simulink library "PiCar_library"  (R2018a)
settings: Solver=VariableStepAuto  StartTime=0.0  StopTime=10.0  RelTol=1e-3
undefined symbols (not defined in the file or in its folder): gray
libraries: visiontextngfix x2, visiontransforms x2, simulink x1, visionanalysis x1, visionstatistics x1, embdlinuxlib x1
settings Model: Creator=Malte  LastModifiedBy=Herib

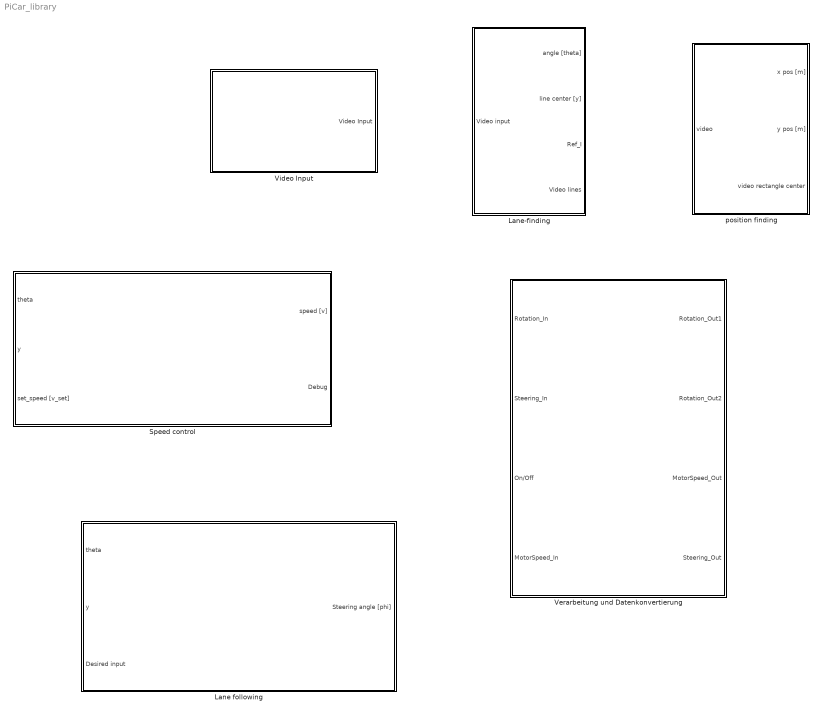
== system PiCar_library ==
  Lane following : Subsystem
  Lane-finding : Subsystem
  Speed control : Subsystem
  Verarbeitung und Datenkonvertierung : Subsystem
  Video Input : Subsystem
  position finding : Subsystem

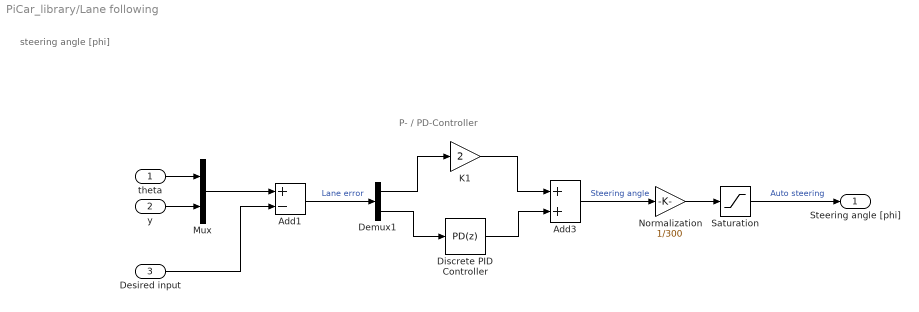
== system PiCar_library/Lane following ==
  note: P- / PD-Controller
  note: steering angle [phi]
  theta : Inport
  y : Inport  Port=2
  Desired input : Inport  Port=3
  Add1 : Sum  Inputs=+-
  Add3 : Sum
  Demux1 : Demux  Outputs=2
  Discrete PID Controller : simulink/Continuous/PID Controller  Controller=PD  TimeDomain=Discrete-time  SampleTime=-1  IntegratorMethod=Forward Euler  FilterMethod=Forward Euler  Form=Parallel  UseFilter=off  ControllerParametersSource=internal  P=18  I=1.5  D=2  N=100  InitialConditionSource=internal  InitialConditionForIntegrator=0  InitialConditionForFilter=0  ExternalReset=none  LimitOutput=off  UpperSaturationLimit=inf  LowerSaturationLimit=-inf  LinearizeAsGain=off  AntiWindupMode=none  Kb=1  TrackingMode=off  Kt=1  PParamMin=[]  PParamMax=[]  IParamMin=[]  IParamMax=[]  DParamMin=[]  DParamMax=[]  NParamMin=[]  NParamMax=[]  KbParamMin=[]  KbParamMax=[]  KtParamMin=[]  KtParamMax=[]  POutMin=[]  POutMax=[]  IOutMin=[]  IOutMax=[]  DOutMin=[]  DOutMax=[]  NOutMin=[]  NOutMax=[]  KbOutMin=[]  KbOutMax=[]  KtOutMin=[]  KtOutMax=[]  IntegratorOutMin=[]  IntegratorOutMax=[]  FilterOutMin=[]  FilterOutMax=[]  SumOutMin=[]  SumOutMax=[]  SumI1OutMin=[]  SumI1OutMax=[]  SumI2OutMin=[]  SumI2OutMax=[]  SumI3OutMin=[]  SumI3OutMax=[]  SumDOutMin=[]  SumDOutMax=[]  SaturationOutMin=[]  SaturationOutMax=[]  IntegratorContinuousStateAttributes=''  IntegratorStateMustResolveToSignalObject=off  IntegratorRTWStateStorageClass=Auto  FilterContinuousStateAttributes=''  FilterStateMustResolveToSignalObject=off  FilterRTWStateStorageClass=Auto  DifferentiatorICPrevScaledInput=0  DifferentiatorOutMin=[]  DifferentiatorOutMax=[]  FilterDiffOutCoefMin=[]  FilterDiffOutCoefMax=[]  SumDenOutMin=[]  SumDenOutMax=[]  SumNumOutMin=[]  SumNumOutMax=[]  ReciprocalOutMin=[]  ReciprocalOutMax=[]  DivideOutMin=[]  DivideOutMax=[]  TunerSelectOption=Transfer Function Based (PID Tuner App)
  K1 : Gain  Gain=2
  Mux : Mux  Inputs=2
  Normalization : Gain  Gain=1/300
  Saturation : Saturate  UpperLimit=1  LowerLimit=-1
  Steering angle [phi] : Outport
  wires:
  K1/1 -> Add3/1
  Demux1/1 -> K1/1
  Add1/1 -> Demux1/1  "Lane error"
  Demux1/2 -> Discrete PID Controller/1
  Discrete PID Controller/1 -> Add3/2
  Add3/1 -> Normalization/1  "Steering angle"
  Saturation/1 -> Steering angle [phi]/1  "Auto steering"
  Normalization/1 -> Saturation/1
  Desired input/1 -> Add1/2
  Mux/1 -> Add1/1
  y/1 -> Mux/2
  theta/1 -> Mux/1

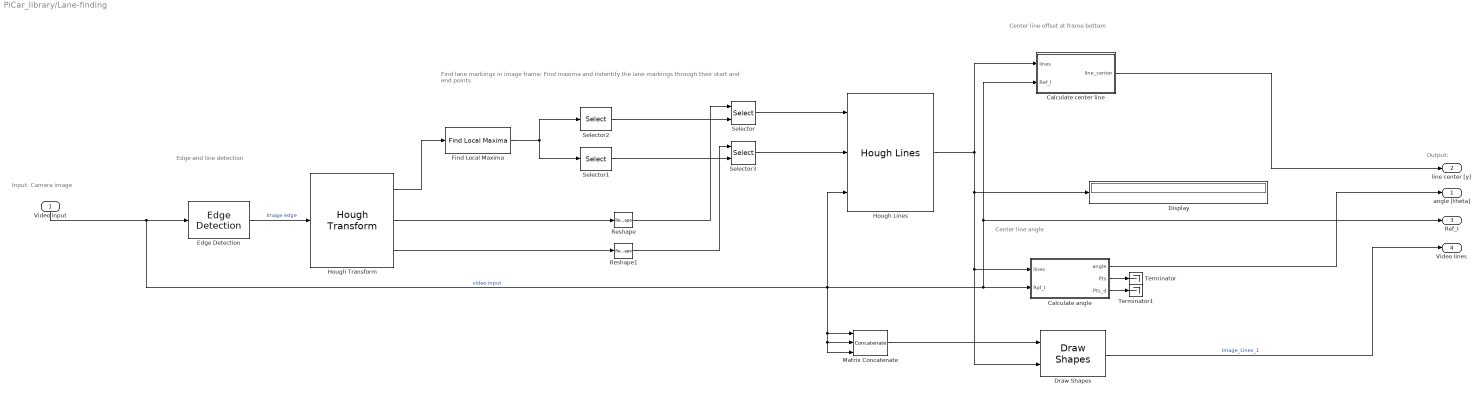
== system PiCar_library/Lane-finding ==
  note: Center line offset at frame bottom
  note: Center line angle
  note: Find lane markings in image frame:
      | Find maxima and indentify the lane markings through their start and end points
  note: Edge and line detection
  note: Input: Camera image
  note: Output:
  Video input : Inport
  Calculate angle : MATLAB Function  TreatAsAtomicUnit=on
  Calculate center line : MATLAB Function  TreatAsAtomicUnit=on
  Display : Display
  Draw Shapes : visiontextngfix/Draw Shapes  shape=Lines  fill=off  lineWidth=1  fillClrSource=Specify via dialog  display=User-specified value  intensity=200  color=[0 0 255]  opacity=0.6  viewport=Entire image  antialiasing=off  inType=Obsolete  imagePorts=One multidimensional signal  prodOutputMode=Binary point scaling  prodOutputWordLength=32  prodOutputFracLength=14  memoryMode=Specify word length  memoryWordLength=16  memoryFracLength=14  roundingMode=Floor  overflowMode=off
      settings: SourceProductName=Computer Vision System Toolbox
  Edge Detection : visionanalysis/Edge Detection  method=Sobel  outputType=Binary image  userDefinedThreshold=off  thresholdSource=Input port  threshold=20  thresholdTuning=4  edgeThinning=off  threshold_canny=[0.25 0.60]  autoPercent=70  sigma=1  roundingMode=Floor  overflowMode=off  prodOutputMode=Binary point scaling  prodOutputWordLength=32  prodOutputFracLength=8  prodOutputSlope=2^-8  accumSlope=2^-8  outputSlope=2^-4
      settings: SourceProductName=Computer Vision System Toolbox  SourceProductBaseCode=VP
  Find Local Maxima : visionstatistics/Find Local Maxima  num_peaks=2  nhood_size=[5 7]  src_thresh=Obsolete9b  src_thresh_inuse=Specify via dialog  threshold=10  inputIsHough=off  dt_peak=uint32  isOutVarDim=on  dt_count=uint32
      settings: SourceProductName=Computer Vision System Toolbox  SourceProductBaseCode=VP
  Hough Lines : visiontransforms/Hough Lines  sineCompMethod=Trigonometric function  thetaRes=pi/180  firstCoeffMode=Specify word length  firstCoeffWordLength=16  firstCoeffFracLength=15  prodOutputMode=Binary point scaling  prodOutputWordLength=32  prodOutputFracLength=16  roundingMode=Nearest  overflowMode=on
      settings: SourceProductName=Computer Vision System Toolbox  SourceProductBaseCode=VP
  Hough Transform : visiontransforms/Hough Transform  theta_res=pi/180  rho_res=1  out_theta_rho=on  outdtmode=double  firstCoeffMode=Binary point scaling  firstCoeffWordLength=16  firstCoeffFracLength=14  secondCoeffMode=Binary point scaling  secondCoeffWordLength=32  secondCoeffFracLength=16  outputMode=Binary point scaling  outputWordLength=16  outputFracLength=0  accumMode=Binary point scaling  accumWordLength=32  accumFracLength=20  prodOutputMode=Binary point scaling  prodOutputWordLength=32  prodOutputFracLength=20  memoryMode=Binary point scaling  memoryWordLength=32  memoryFracLength=16  roundingMode=Nearest  overflowMode=on
      settings: SourceProductName=Computer Vision System Toolbox  SourceProductBaseCode=VP
  Matrix Concatenate : Concatenate  NumInputs=3  Mode=Multidimensional array  ConcatenateDimension=3
  Reshape : Reshape
  Reshape1 : Reshape
  Selector : Selector  IndexOptions=Index vector (port)  Indices=[1 3]  OutputSizes=1
  Selector1 : Selector  NumberOfDimensions=2  InputPortWidth=3  IndexOptions=Select all,Index vector (dialog)  Indices=[1 3],2  OutputSizes=1,1
  Selector2 : Selector  NumberOfDimensions=2  InputPortWidth=3  IndexOptions=Select all,Index vector (dialog)  Indices=[1 3],1  OutputSizes=1,1
  Selector3 : Selector  IndexOptions=Index vector (port)  Indices=[1 3]  OutputSizes=1
  Terminator : Terminator
  Terminator1 : Terminator
  angle [theta] : Outport
  line center [y] : Outport  Port=2
  Ref_I : Outport  Port=3
  Video lines : Outport  Port=4
  wires:
  Calculate angle/2(Pts) -> Terminator/1
  Calculate angle/3(Pts_d) -> Terminator1/1
  Edge Detection/1 -> Hough Transform/1  "Image edge"
  Video input/1 -> Calculate angle/2(Ref_I), Calculate center line/2(Ref_I), Ref_I/1, Hough Lines/3, Matrix Concatenate/1, Matrix Concatenate/2, Matrix Concatenate/3, Edge Detection/1  "video input"
  Hough Transform/2 -> Reshape/1
  Hough Transform/3 -> Reshape1/1
  Hough Transform/1 -> Find Local Maxima/1
  Selector1/1 -> Selector3/2
  Selector2/1 -> Selector/2
  Find Local Maxima/1 -> Selector2/1, Selector1/1
  Selector/1 -> Hough Lines/1
  Reshape/1 -> Selector/1
  Selector3/1 -> Hough Lines/2
  Reshape1/1 -> Selector3/1
  Matrix Concatenate/1 -> Draw Shapes/1
  Calculate angle/1(angle) -> angle [theta]/1
  Draw Shapes/1 -> Video lines/1  "Image_Lines_1"
  Hough Lines/1 -> Calculate center line/1(lines), Display/1, Draw Shapes/2, Calculate angle/1(lines)
  Calculate center line/1(line_center) -> line center [y]/1

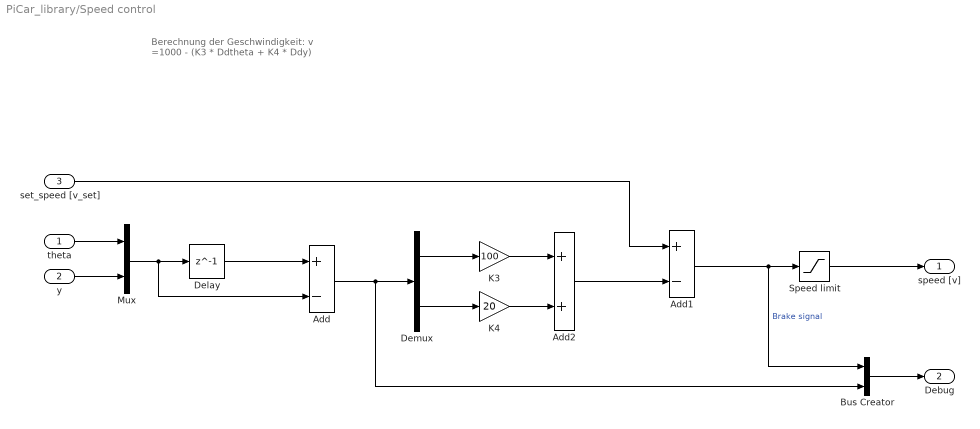
== system PiCar_library/Speed control ==
  note: Berechnung der Geschwindigkeit:
      |
      | v =1000 - (K3 * Ddtheta + K4 * Ddy)
  theta : Inport
  y : Inport  Port=2
  set_speed [v_set] : Inport  Port=3
  Add : Sum  Inputs=+-
  Add1 : Sum  Inputs=+-
  Add2 : Sum
  Bus Creator : BusCreator  Inputs=2
  Delay : Delay  DelayLength=1  InitialCondition=0
  Demux : Demux  Outputs=2
  K3 : Gain  Gain=100
  K4 : Gain  Gain=20
  Mux : Mux  Inputs=2
  Speed limit : Saturate  UpperLimit=0.4  LowerLimit=0
  speed [v] : Outport
  Debug : Outport  Port=2
  wires:
  Mux/1 -> Add/2, Delay/1
  Delay/1 -> Add/1
  Add/1 -> Bus Creator/2, Demux/1
  Demux/1 -> K3/1
  Demux/2 -> K4/1
  Add2/1 -> Add1/2
  Add1/1 -> Bus Creator/1, Speed limit/1  "Brake signal"
  set_speed [v_set]/1 -> Add1/1
  K4/1 -> Add2/2
  K3/1 -> Add2/1
  Bus Creator/1 -> Debug/1
  y/1 -> Mux/2
  theta/1 -> Mux/1
  Speed limit/1 -> speed [v]/1

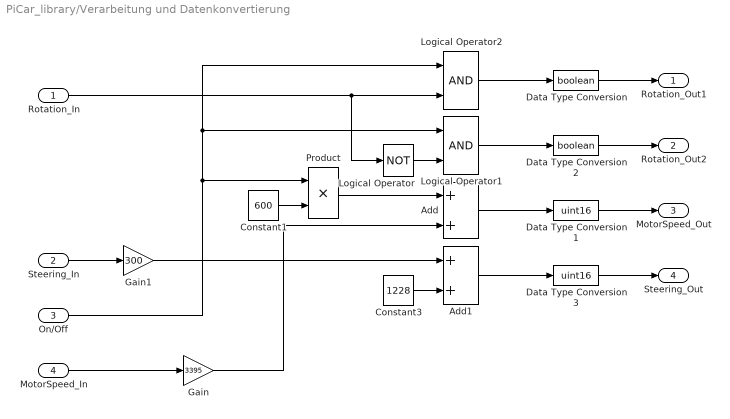
== system PiCar_library/Verarbeitung und Datenkonvertierung ==
  Rotation_In : Inport
  Steering_In : Inport  Port=2
  On/Off : Inport  Port=3
  MotorSpeed_In : Inport  Port=4
  Add : Sum
  Add1 : Sum
  Constant1 : Constant  Value=600
  Constant3 : Constant  Value=1228  OutMin=819  OutMax=1638
  Data Type Conversion : DataTypeConversion  OutDataTypeStr=boolean
  Data Type Conversion1 : DataTypeConversion  OutDataTypeStr=uint16
  Data Type Conversion2 : DataTypeConversion  OutDataTypeStr=boolean
  Data Type Conversion3 : DataTypeConversion  OutDataTypeStr=uint16
  Gain : Gain  Gain=3395
  Gain1 : Gain  Gain=300
  Logical Operator : Logic  Operator=NOT  AllPortsSameDT=off  OutDataTypeStr=boolean
  Logical Operator1 : Logic  AllPortsSameDT=off  OutDataTypeStr=boolean
  Logical Operator2 : Logic  AllPortsSameDT=off  OutDataTypeStr=boolean
  Product : Product
  Rotation_Out1 : Outport
  Rotation_Out2 : Outport  Port=2
  MotorSpeed_Out : Outport  Port=3
  Steering_Out : Outport  Port=4
  wires:
  Logical Operator1/1 -> Data Type Conversion2/1
  Logical Operator2/1 -> Data Type Conversion/1
  Logical Operator/1 -> Logical Operator1/2
  On/Off/1 -> Logical Operator1/1, Logical Operator2/1, Product/1
  Constant3/1 -> Add1/2
  Rotation_In/1 -> Logical Operator/1, Logical Operator2/2
  Add/1 -> Data Type Conversion1/1
  Add1/1 -> Data Type Conversion3/1
  Constant1/1 -> Product/2
  Product/1 -> Add/1
  Data Type Conversion1/1 -> MotorSpeed_Out/1
  Data Type Conversion3/1 -> Steering_Out/1
  Data Type Conversion2/1 -> Rotation_Out2/1
  MotorSpeed_In/1 -> Gain/1
  Data Type Conversion/1 -> Rotation_Out1/1
  Steering_In/1 -> Gain1/1
  Gain/1 -> Add/2
  Gain1/1 -> Add1/1

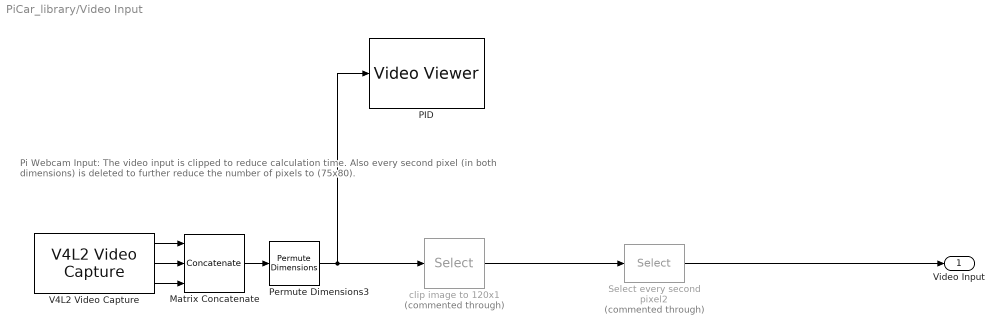
== system PiCar_library/Video Input ==
  note: Pi Webcam Input:
      | The video input is clipped to reduce calculation time. Also every second pixel (in both dimensions) is deleted to further reduce the number of pixels
      | to (75x80).
  Matrix Concatenate : Concatenate  NumInputs=3  Mode=Multidimensional array  ConcatenateDimension=3
  PID : VideoViewer  colormapValue=gray(256)  FigPos=[1 1038 1920 938]  OpenAtMdlStart=off
  Permute Dimensions3 : PermuteDimensions  Order=[2,1,3]
  Select every second pixel2 : Selector  Commented=through  NumberOfDimensions=2  InputPortWidth=3  IndexOptions=Select all,Index vector (dialog)  Indices=[1:2:80],[1:2:160]  OutputSizes=1,1
  V4L2 Video Capture : embdlinuxlib/V4L2 Video Capture  m_devName='/dev/video0'  roi=[0, 0, 640, 480]  imSizeSelection=320x240  imSize=[640, 480]  pixelFormat=RGB  pixelOrder=Planar  sampleTime=1/10  simOutput=Colorbars  blockPlatform=Raspberry Pi
      settings: SourceProductName=Simulink Support Package for Raspberry Pi Hardware  SourceProductBaseCode=RASPPI
  clip image to 120x1 : Selector  Commented=through  NumberOfDimensions=2  InputPortWidth=3  IndexOptions=Index vector (dialog),Index vector (dialog)  Indices=[150:1:210],[1:2:320]  OutputSizes=1,1
  Video Input : Outport
  wires:
  Permute Dimensions3/1 -> PID/1, clip image to 120x1/1
  clip image to 120x1/1 -> Select every second pixel2/1
  V4L2 Video Capture/2 -> Matrix Concatenate/2
  V4L2 Video Capture/3 -> Matrix Concatenate/3
  Select every second pixel2/1 -> Video Input/1
  V4L2 Video Capture/1 -> Matrix Concatenate/1
  Matrix Concatenate/1 -> Permute Dimensions3/1

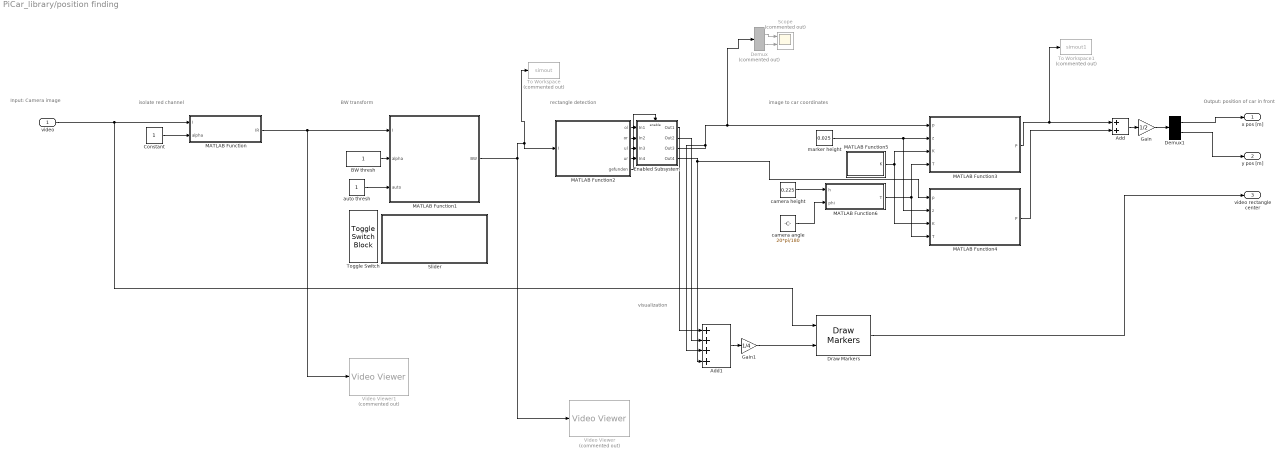
== system PiCar_library/position finding ==
  note: Input: Camera image
  note: Output: position of car in front
  note: isolate red channel
  note: BW transform
  note: rectangle detection
  note: image to car coordinates
  note: visualization
  video : Inport
  Add : Sum  Inputs=2
  Add1 : Sum  Inputs=4
  BW thresh : Constant
  Constant : Constant
  Demux : Demux  Commented=on  Outputs=2
  Demux1 : Demux  Outputs=2
  Draw Markers : visiontextngfix/Draw Markers  shape=Circle  size=3  fill=off  fillClrSource=Specify via dialog  display=Black  intensity=200  color=[200 255 100]  opacity=0.6  viewport=Entire image  antialiasing=off  inType=Obsolete  imagePorts=One multidimensional signal  prodOutputMode=Binary point scaling  prodOutputWordLength=32  prodOutputFracLength=14  memoryMode=Specify word length  memoryWordLength=16  memoryFracLength=15  roundingMode=Floor  overflowMode=off
      settings: SourceProductName=Computer Vision System Toolbox  SourceProductBaseCode=VP
  Enabled Subsystem : Subsystem  TreatAsAtomicUnit=on
  Gain : Gain  Gain=1/2
  Gain1 : Gain  Gain=1/4
  MATLAB Function : MATLAB Function  TreatAsAtomicUnit=on
  MATLAB Function1 : MATLAB Function  TreatAsAtomicUnit=on
  MATLAB Function2 : MATLAB Function  TreatAsAtomicUnit=on
  MATLAB Function3 : MATLAB Function  TreatAsAtomicUnit=on
  MATLAB Function4 : MATLAB Function  TreatAsAtomicUnit=on
  MATLAB Function5 : MATLAB Function  TreatAsAtomicUnit=on
  MATLAB Function6 : MATLAB Function  TreatAsAtomicUnit=on
  Scope : Scope  Commented=on  NumInputPorts=2
  Slider : Subsystem  DialogController=hmiCreateDDGDialog  IsWebBlock=on  mask(MWDashboardBlock){webBlockId=af7e4ece-416e-4c7c-9f64-5e96a6a09053, webBlockType=slider, ShowInLibBrowser=on, ShowInitialText=on, HMISrcModelName=PiCar_library}
      mask prompts: webBlockId "WebBlock Id"; webBlockType "WebBlock Type"; HMISrcModelName "Source Model"
      mask help: SimulinkHMI:dialogs:SliderDialogDesc
      mask Help: helpview([docroot '/mapfiles/simulink.map'], 'hmi_slider')
      mask Display:
      | if strcmp(get_param(bdroot(gcb),'BlockDiagramType'), 'library')
      |     image([(matlabroot) '/toolbox/simulink/hmi/icons/Slider.png']);
      | end
  To Workspace : ToWorkspace  Commented=on  VariableName=simout  SaveFormat=Structure  SampleTime=-1
      settings: MaxDataPoints=1
  To Workspace1 : ToWorkspace  Commented=on  VariableName=simout1  SaveFormat=Timeseries  SampleTime=-1
  Toggle Switch : ToggleSwitchBlock  WebBlockId=151
      settings: Values={{'Off', 'On'}, [0 1]}
  Video Viewer : VideoViewer  Commented=on  FigPos=[2041 741 418 304]
  Video Viewer1 : VideoViewer  Commented=on  FigPos=[2041 741 418 304]
  auto thresh : Constant
  camera angle : Constant  Value=20*pi/180
  camera height : Constant  Value=0.225
  marker height : Constant  Value=0.025
  x pos [m] : Outport
  y pos [m] : Outport  Port=2
  video rectangle center : Outport  Port=3
  wires:
  Constant/1 -> MATLAB Function/2(alpha)
  MATLAB Function/1(IR) -> Video Viewer1/1, MATLAB Function1/1(I)
  BW thresh/1 -> MATLAB Function1/2(alpha)
  auto thresh/1 -> MATLAB Function1/3(auto)
  MATLAB Function1/1(BW) -> To Workspace/1, MATLAB Function2/1(I), Video Viewer/1
  MATLAB Function3/1(P) -> To Workspace1/1, Add/1
  Add/1 -> Gain/1
  Add1/1 -> Gain1/1
  Enabled Subsystem/1(Out1) -> Add1/1
  Enabled Subsystem/2(Out2) -> Add1/2
  Gain1/1 -> Draw Markers/2
  video/1 -> Draw Markers/1, MATLAB Function/1(I)
  Draw Markers/1 -> video rectangle center/1
  MATLAB Function4/1(P) -> Add/2
  marker height/1 -> MATLAB Function4/2(z), MATLAB Function3/2(z)
  MATLAB Function5/1(K) -> MATLAB Function4/3(K), MATLAB Function3/3(K)
  MATLAB Function6/1(T) -> MATLAB Function4/4(T), MATLAB Function3/4(T)
  camera height/1 -> MATLAB Function6/1(h)
  camera angle/1 -> MATLAB Function6/2(phi)
  Demux1/1 -> x pos [m]/1
  MATLAB Function2/5(gefunden) -> Enabled Subsystem/Enable
  MATLAB Function2/1(ol) -> Enabled Subsystem/1(In1)
  MATLAB Function2/2(or) -> Enabled Subsystem/2(In2)
  MATLAB Function2/3(ul) -> Enabled Subsystem/3(In3)
  MATLAB Function2/4(ur) -> Enabled Subsystem/4(In4)
  Demux/2 -> Scope/2
  Demux/1 -> Scope/1
  Enabled Subsystem/3(Out3) -> MATLAB Function3/1(p), Demux/1, Add1/3
  Enabled Subsystem/4(Out4) -> MATLAB Function4/1(p), Add1/4
  Gain/1 -> Demux1/1
  Demux1/2 -> y pos [m]/1

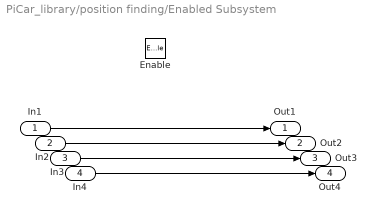
== system PiCar_library/position finding/Enabled Subsystem ==
  In1 : Inport
  In2 : Inport  Port=2
  In3 : Inport  Port=3
  In4 : Inport  Port=4
  Enable : EnablePort  StatesWhenEnabling=reset  PropagateVarSize=During execution
  Out1 : Outport
  Out2 : Outport  Port=2
  Out3 : Outport  Port=3
  Out4 : Outport  Port=4
  wires:
  In1/1 -> Out1/1
  In2/1 -> Out2/1
  In3/1 -> Out3/1
  In4/1 -> Out4/1

== system PiCar_library/position finding/Slider ==

== matlab function PiCar_library/Lane-finding/Calculate angle ==
  data: lines input; angle output; Pts output; Pts_d output; Ref_I input
function [angle, Pts, Pts_d] = angle(lines, Ref_I)

IMAGE_SIZE = size(Ref_I);
IMAGE_HEIGHT = IMAGE_SIZE(1);
IMAGE_WIDTH = IMAGE_SIZE(2);
points = zeros(2,4);

% Sorting the lines
if double(lines(1,1)) < double(lines(2,1))
    points(1,:) = lines(1,:);
    points(2,:) = lines(2,:);
else
    points(1,:) = lines(2,:);
    points(2,:) = lines(1,:);
end

% Calculate the lane center, top and bottom
x_center = double((points(1,:) + points(2,:))/2);

% Calculate the angle of the centerline: 0 -> vertical
angle = atan((x_center(3) - x_center(1))/IMAGE_HEIGHT);

% Auxilliary lines
Pts = int32([x_center(1), 1, x_center(3), 75]);
Pts_d = int32([IMAGE_WIDTH/2, 1, IMAGE_WIDTH/2, 75]);

% angles = atan2d(double((lines(:,1) - lines(:,3))), -double(lines(:,2) - lines(:,4)));

== matlab function PiCar_library/Lane-finding/Calculate center line ==
  data: lines input; line_center output; Ref_I input
function line_center = center(lines, Ref_I)

IMAGE_SIZE = size(Ref_I);
IMAGE_HEIGHT = IMAGE_SIZE(1);
IMAGE_WIDTH = IMAGE_SIZE(2);
points = zeros(2,4);

% Sorting the lines
if double(lines(1,1)) < double(lines(2,1))
    points(1,:) = lines(1,:);
    points(2,:) = lines(2,:);
else
    points(1,:) = lines(2,:);
    points(2,:) = lines(1,:);
end

% Calculate the lane center, top and bottom
x_center = double((points(1,:) + points(2,:))/2);

% Output the lane center at the bottom of the picture
line_center = x_center(3);

== matlab function PiCar_library/position finding/MATLAB Function ==
  data: I input; IR output; alpha input
function IR = isolate_red(I, alpha)
    IR = I(:,:,1) - alpha*I(:,:,2) - alpha*I(:,:,3);
end

== matlab function PiCar_library/position finding/MATLAB Function1 ==
  data: I input; BW output; alpha input; auto input
function BW = BW_im(I, alpha, auto)
    if(auto)
        BW = imbinarize(I);
    else
        BW = imbinarize(I,alpha);
    end
end

== matlab function PiCar_library/position finding/MATLAB Function2 ==
  data: I input; ol output; or output; ul output; ur output; gefunden output
function [ol, or, ul, ur, gefunden]  = finderechteck(I)
%fuer die Aufloesung 160x120
%findet koordinaten der Ecken des rechteckes im Bild
%IGr=rgb2gray(I);
%IG=imgaussfilt(IGr,5);
%I=max(I(:,:,1),0); %rot vorheben
%imshow([I(:,:,1) I(:,:,2); I(:,:,3) I(:,:,1)-0.5*I(:,:,2)-0.5*I(:,:,3)]);
%imshow(I);
x1=floor(size(I,2)/2);
y1=floor(size(I,1)/2);
iteration=1;
schrittgroesse=10;
%imshow(I)
%hold on;
finished=false;
[imagepoints]=rechteck(I,x1,y1);
if imagepoints(1)~=-1
    finished=true;
end

%spiralfoermiges durchlaufen zur quadratsuche
while(finished==false)
    
    for i=1:iteration
        x1=x1+schrittgroesse;
        [imagepoints]=rechteck(I,x1,y1);
        if imagepoints(1)~=-1
            finished=true;
            break;
        end
    end
    
    if finished~=true
        for i=1:iteration
            if (y1-schrittgroesse>1)
                y1=y1-schrittgroesse;
            else
                finished=true;
            end
            [imagepoints]=rechteck(I,x1,y1);
            if imagepoints(1)~=-1
                finished=true;
                
                break;
            end
        end
    end
    
    
    if finished~=true
        iteration=iteration+1;
        for i=1:iteration
            x1=x1-schrittgroesse;
            [imagepoints]=rechteck(I,x1,y1);
            if imagepoints(1)~=-1
                finished=true;
                
                break;
            end
        end
    end
    if finished~=true
        for i=1:iteration
            if (y1+schrittgroesse<size(I,1))
                y1=y1+schrittgroesse;
            else
                finished=true;
            end
            [imagepoints]=rechteck(I,x1,y1);
            if imagepoints(1)~=-1
                finished=true;
                
                break;
            end
        end
        
        iteration=iteration+1;
        
    end
end

ol = imagepoints(1,:);
or = imagepoints(2,:);
ul = imagepoints(3,:);
ur = imagepoints(4,:);
gefunden = imagepoints(1,1) ~= -1;

end


function [imagepoints]=rechteck(BW,x1,y1)

Farbe=1;

seitenabstand=5;



x=x1;
y=y1;
while (BW(y,x)==Farbe)
    
    if y>2
        y=y-1;
    else
        break;
    end
end

b1=y;

x=x1;
y=y1;
while (BW(y,x)==Farbe)
    
    if y<size(BW,1)
        y=y+1;
    else
        break;
    end
end

b2=y;

ym=floor((b1+b2)/2);

x=x1;
y=ym;

while (BW(y,x)==Farbe)
    
    if x<size(BW,2)
        x=x+1;
    else
        break;
    end
end

xr=x-seitenabstand;

x=x1;
y=ym;


while (BW(y,x)==Farbe)
    
    if x>1
        x=x-1;
    else
        break;
    end
end

xl=x+seitenabstand;



x2=xl;
y2=ym;

x=x2;
y=y2;
while (BW(y,x)==Farbe)
    
    if y>2
        y=y-1;
    else
        break;
    end
end

b1=y;

x=x2;
y=y2;
while (BW(y,x)==Farbe)
    
    if y<size(BW,1)
        y=y+1;
    else
        break;
    end
end

b2=y;

xol=xl-seitenabstand;
xul=xl-seitenabstand;
yol=b1;
yul=b2;


x3=xr;
y3=ym;

x=x3;
y=y3;
while (BW(y,x)==Farbe)
    
    if y>2
        y=y-1;
    else
        break;
    end
end

b1=y;

x=x3;
y=y3;
while (BW(y,x)==Farbe)
    
    if y<size(BW,1)
        y=y+1;
    else
        break;
    end
end

b2=y;

xor=xr+seitenabstand;
xur=xr+seitenabstand;
yor=b1;
yur=b2;

l_links=yul-yol;
l_rechts=yur-yor;
l_mitte=xr-xl;

%sinnvolle quadratdimensionen?
if (l_links>1.3*l_rechts || l_rechts>1.3*l_links ||...
        l_links>1.3*l_mitte || l_mitte>1.3*l_links ...
        ||  max((ym-yol)/(ym-yor),(yul-ym)/(yur-ym))>1.3...
        ||l_mitte<5)
    %plot(x1,y1,'o');
    %plot(x1,y1,'+');
    %plot ([xr xr],[yor yur]);
    %plot ([xl xl],[yol yul]);
    %plot ([xl xr],[ym ym]);
    imagepoints=[-1 yol; xor yor;xul yul; xur yur];
else %sinvolles quadrat gefunden
    %plot(x1,y1,'+');
    imagepoints=[xol yol; xor yor;xul yul; xur yur];
end

end

== matlab function PiCar_library/position finding/MATLAB Function3 ==
  data: p input; P output; z input; K input; T input
function P = pixel2car(p,z,K,T)
% PIXEL2WORLD calculates the world coordinates of p
%   p: pixel coordinates
%   z: heigt of point in world coordinates
%   K: intrinsic camera matrix
%   T: homogeneous transformation matrix of camera to world pose
%
%   P: world coordinates (column vector)
p = p(:);
g = K\[p;1];
lambda = T(3,1:3)*g/(z-T(3,4));
P = T(1:3,:)*[g/lambda; 1];

end

== matlab function PiCar_library/position finding/MATLAB Function4 ==
  data: p input; P output; z input; K input; T input
function P = pixel2car(p,z,K,T)
% PIXEL2WORLD calculates the world coordinates of p
%   p: pixel coordinates
%   z: heigt of point in world coordinates
%   K: intrinsic camera matrix
%   T: homogeneous transformation matrix of camera to world pose
%
%   P: world coordinates (column vector)
p = p(:);
g = K\[p;1];
lambda = T(3,1:3)*g/(z-T(3,4));
P = T(1:3,:)*[g/lambda; 1];

end

== matlab function PiCar_library/position finding/MATLAB Function5 ==
  data: K output
function K = intrinsic_mat()
% PiCam, resultion 2464x3280:
n = 3280;
K = 1.0e+03 * ...
   [2.5966         0         0; ...
         0    2.6037         0; ...
    1.6534    1.2445    0.0010];

% Scaling to adjust resolution:
x_pixels = 320;



% % surface rear camera, resolution 2448 3264
% n = 3264;
% K = 1.0e+03 * ...
%    [2.6081         0         0; ...
%          0    2.5796         0; ...
%     1.6621    1.1589    0.0010];
% K(:,1:2) = K(:,1:2)*480/2448;
% 
% % Scaling to adjust resolution:
% x_pixels = 640;

K(:,1:2) = K(:,1:2)*x_pixels/n;
K = K';

end

== matlab function PiCar_library/position finding/MATLAB Function6 ==
  data: h input; T output; phi input
function T = world2cam(h, phi)
% calculates the homogeneous transormationf matrix of the camera's pose
%   h:      height of the camera above ground
%   phi:    angle of camera around y axis

T = [   0   -sin(phi)   cos(phi)    0;   ...
       -1           0          0    0;   ...
        0   -cos(phi)  -sin(phi)    h;   ...
        0           0          0    1];

end
